simulink model "Combined_electrolyzer_simulink"  (R2022a)
settings: Solver=FixedStepAuto  StartTime=0.0  StopTime=1000  FixedStep=1  RelTol=1e-3
settings Model: Creator=Anupp  LastModifiedBy=Anupp

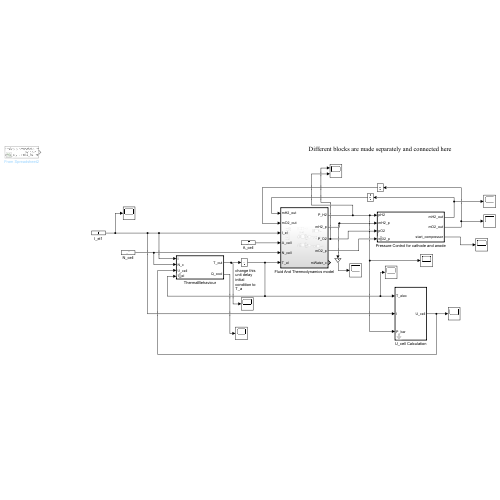
[thumbnail: Simulink's stored preview of the top-level diagram]
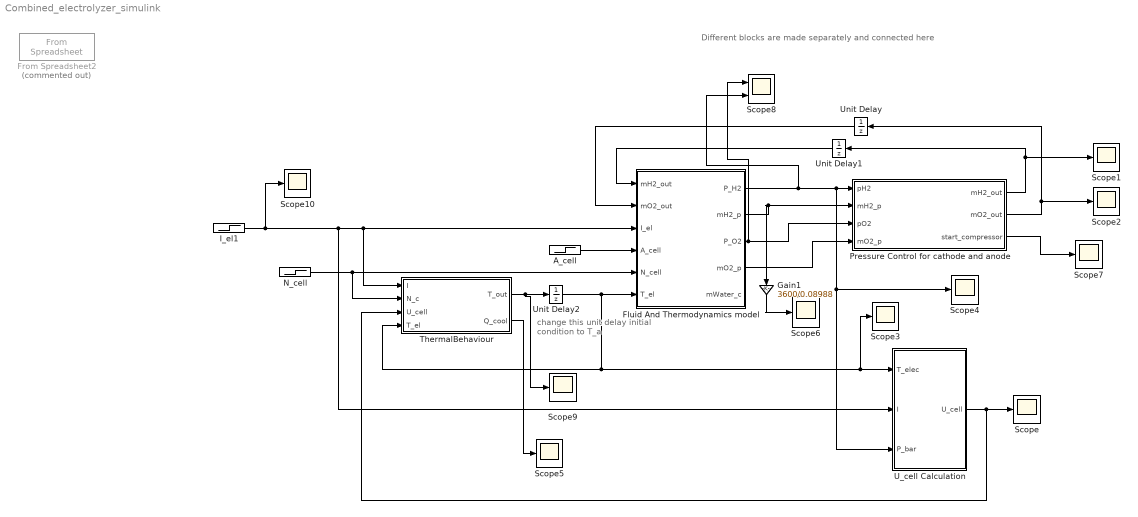
== system Combined_electrolyzer_simulink ==
  note: Different blocks are made separately and connected here
  note: change this unit delay initial condition to T_a
  A_cell : Step  Time=0  After=37.476  SampleTime=0
  Fluid And Thermodynamics model : Subsystem  TreatAsAtomicUnit=on
  From Spreadsheet2 : FromSpreadsheet  Commented=on  FileName=E:\tintan\Matlab alakaline electrolysis new\data test\down_dynamic_halved.csv  SheetName=down_dynamic_halved
  Gain1 : Gain  Gain=3600/0.08988
  I_el1 : Step  Time=0  After=4567.5  SampleTime=0
  N_cell : Step  Time=0  After=326  SampleTime=0
  Pressure Control for cathode and anode : Subsystem  TreatAsAtomicUnit=on  mask{P_nominal=16e+05}
      mask prompts: P_nominal "Nominal Electrolyzer Pressure"
  Scope{,1..7,9..10} (10 alike) : Scope
  Scope8 : Scope  NumInputPorts=2
  ThermalBehaviour : Subsystem  TreatAsAtomicUnit=on  mask{E_tn=1.476, T_a=298, R_t=0.4441, C_t=1.6824e+05, T_nominal=353}
      mask prompts: E_tn "Thermo-neutral voltage (E_tn)"; T_a "Ambient Temperature (kelvin)"; R_t "Thermal Resistance"; C_t "Thermal Capacitance"; T_nominal "Nominal Temperature (kelvin)"
  U_cell Calculation : Subsystem  TreatAsAtomicUnit=on  mask{A=26600, r1=0.8, r2=-0.00763, t1=20, t2=0.1, t3=3.5e+05, s=0.1795, C=0.25}
      mask prompts: A "Area"; r1 "r1 for U_ohm"; r2 "r2 for U_ohm"; t1 "t1 for U_act"; t2 "t2 for U_act"; t3 "t3 for U_act"; s "s for U_act"; C "Concentration by weight (decimal)"
      mask DialogControl DescTextVar Prompt: Put all values in terms in Metres only or Cm only. Also check if U_act variables is for Log or Ln (change accordingly inside the mask). Also, use concentration value as decimal (for eg. use 0.25, don't use 25 percent).
  Unit Delay : UnitDelay  SampleTime=-1  HasFrameUpgradeWarning=on
  Unit Delay1 : UnitDelay  SampleTime=-1  HasFrameUpgradeWarning=on
  Unit Delay2 : UnitDelay  InitialCondition=298  SampleTime=-1  HasFrameUpgradeWarning=on
  wires:
  Fluid And Thermodynamics model/1(P_H2) -> Scope8/2, Scope4/1, U_cell Calculation/3(P_bar), Pressure Control for cathode and anode/1(pH2)
  Fluid And Thermodynamics model/3(P_O2) -> Scope8/1, Pressure Control for cathode and anode/3(pO2)
  Fluid And Thermodynamics model/4(mO2_p) -> Pressure Control for cathode and anode/4(mO2_p)
  Pressure Control for cathode and anode/1(mH2_out) -> Scope1/1, Unit Delay1/1
  Pressure Control for cathode and anode/2(mO2_out) -> Scope2/1, Unit Delay/1
  Unit Delay1/1 -> Fluid And Thermodynamics model/1(mH2_out)
  Unit Delay/1 -> Fluid And Thermodynamics model/2(mO2_out)
  ThermalBehaviour/1(T_out) -> Scope9/1, Unit Delay2/1
  U_cell Calculation/1(U_cell) -> Scope/1, ThermalBehaviour/3(U_cell)
  Unit Delay2/1 -> Scope3/1, U_cell Calculation/1(T_elec), ThermalBehaviour/4(T_el), Fluid And Thermodynamics model/6(T_el)
  I_el1/1 -> U_cell Calculation/2(I), ThermalBehaviour/1(I), Fluid And Thermodynamics model/3(I_el), Scope10/1
  A_cell/1 -> Fluid And Thermodynamics model/4(A_cell)
  N_cell/1 -> ThermalBehaviour/2(N_c), Fluid And Thermodynamics model/5(N_cell)
  ThermalBehaviour/2(Q_cool) -> Scope5/1
  Pressure Control for cathode and anode/3(start_compressor) -> Scope7/1
  Fluid And Thermodynamics model/2(mH2_p) -> Pressure Control for cathode and anode/2(mH2_p), Gain1/1
  Gain1/1 -> Scope6/1

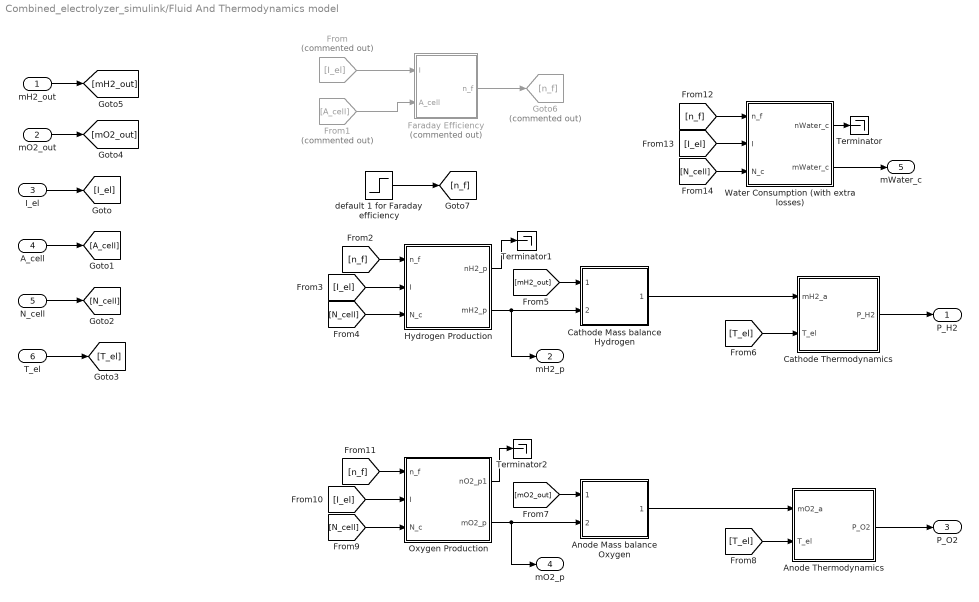
== system Combined_electrolyzer_simulink/Fluid And Thermodynamics model ==
  mH2_out : Inport
  mO2_out : Inport  Port=2
  I_el : Inport  Port=3
  A_cell : Inport  Port=4
  N_cell : Inport  Port=5
  T_el : Inport  Port=6
  Anode Mass balance Oxygen : Subsystem
  Anode Thermodynamics : Subsystem  mask{V=0.001}
      mask prompts: V "Anode Volume"
  Cathode Mass balance Hydrogen : Subsystem
  Cathode Thermodynamics : Subsystem  mask{V=0.001}
      mask prompts: V "Cathode Volume"
  Faraday Efficiency : Subsystem  Commented=on  mask{a1=0, a2=0, a3=0}
      mask DialogControl DescTextVar Prompt: Define Faraday's efficiency parameters for alkaline electrolyser
  From : From  Commented=on  GotoTag=I_el
  From1 : From  Commented=on  GotoTag=A_cell
  Goto6 : Goto  Commented=on  GotoTag=n_f
  Hydrogen Production : Subsystem
  Oxygen Production : Subsystem
  Terminator : Terminator
  Terminator1 : Terminator
  Terminator2 : Terminator
  Water Consumption (with extra losses) : Subsystem
  default 1 for Faraday efficiency : Step  Time=0  After=0.86  SampleTime=0
  P_H2 : Outport
  mH2_p : Outport  Port=2
  P_O2 : Outport  Port=3
  mO2_p : Outport  Port=4
  mWater_c : Outport  Port=5
  wires:
  From1/1 -> Faraday Efficiency/2(A_cell)
  From/1 -> Faraday Efficiency/1(I)
  Cathode Mass balance Hydrogen/1(mH2_a) -> Cathode Thermodynamics/1(mH2_a)
  [n_f] -> Hydrogen Production/1(n_f)
  T_el/1 -> [T_el]
  [I_el] -> Water Consumption (with extra losses)/2(I)
  Hydrogen Production/2(mH2_p) -> mH2_p/1, Cathode Mass balance Hydrogen/2(mH2_p)
  N_cell/1 -> [N_cell]
  I_el/1 -> [I_el]
  [n_f] -> Oxygen Production/1(n_f)
  mO2_out/1 -> [mO2_out]
  Water Consumption (with extra losses)/2(mWater_c) -> mWater_c/1
  A_cell/1 -> [A_cell]
  mH2_out/1 -> [mH2_out]
  [I_el] -> Oxygen Production/2(I)
  [N_cell] -> Oxygen Production/3(N_c)
  [mH2_out] -> Cathode Mass balance Hydrogen/1(mH2_out)
  [N_cell] -> Hydrogen Production/3(N_c)
  Oxygen Production/2(mO2_p) -> mO2_p/1, Anode Mass balance Oxygen/2(mO2_p)
  [I_el] -> Hydrogen Production/2(I)
  Faraday Efficiency/1(n_f) -> Goto6/1
  [T_el] -> Cathode Thermodynamics/2(T_el)
  [N_cell] -> Water Consumption (with extra losses)/3(N_c)
  [n_f] -> Water Consumption (with extra losses)/1(n_f)
  [T_el] -> Anode Thermodynamics/2(T_el)
  Anode Mass balance Oxygen/1(mO2_a) -> Anode Thermodynamics/1(mO2_a)
  [mO2_out] -> Anode Mass balance Oxygen/1(mO2_out)
  Cathode Thermodynamics/1(P_H2) -> P_H2/1
  Anode Thermodynamics/1(P_O2) -> P_O2/1
  Water Consumption (with extra losses)/1(nWater_c) -> Terminator/1
  Hydrogen Production/1(nH2_p) -> Terminator1/1
  Oxygen Production/1(nO2_p1) -> Terminator2/1
  default 1 for Faraday efficiency/1 -> [n_f]

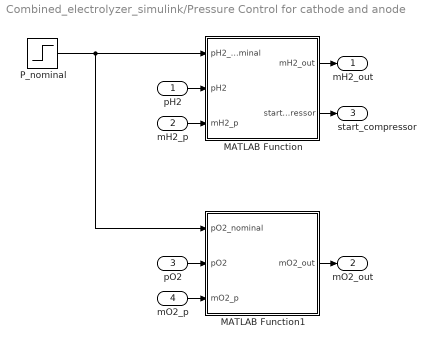
== system Combined_electrolyzer_simulink/Pressure Control for cathode and anode ==
  pH2 : Inport
  mH2_p : Inport  Port=2
  pO2 : Inport  Port=3
  mO2_p : Inport  Port=4
  MATLAB Function : MATLAB Function  TreatAsAtomicUnit=on
  MATLAB Function1 : MATLAB Function  TreatAsAtomicUnit=on
  P_nominal : Step  Time=0  After=P_nominal  SampleTime=0
  mH2_out : Outport
  mO2_out : Outport  Port=2
  start_compressor : Outport  Port=3
  wires:
  P_nominal/1 -> MATLAB Function1/1(pO2_nominal), MATLAB Function/1(pH2_nominal)
  mH2_p/1 -> MATLAB Function/3(mH2_p)
  MATLAB Function/2(start_compressor) -> start_compressor/1
  MATLAB Function/1(mH2_out) -> mH2_out/1
  pH2/1 -> MATLAB Function/2(pH2)
  MATLAB Function1/1(mO2_out) -> mO2_out/1
  mO2_p/1 -> MATLAB Function1/3(mO2_p)
  pO2/1 -> MATLAB Function1/2(pO2)

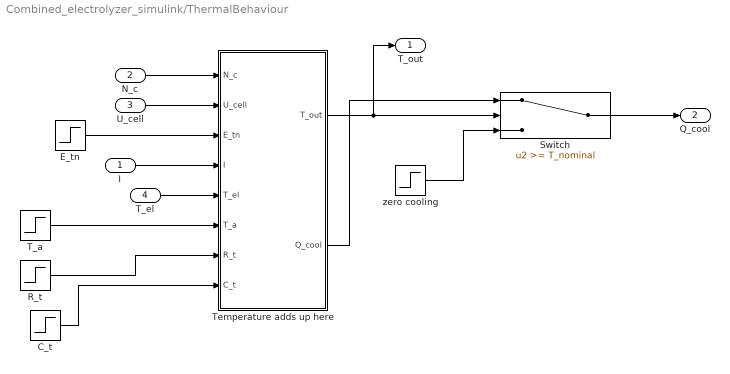
== system Combined_electrolyzer_simulink/ThermalBehaviour ==
  I : Inport
  N_c : Inport  Port=2
  U_cell : Inport  Port=3
  T_el : Inport  Port=4
  C_t : Step  Time=0  After=C_t  SampleTime=0
  E_tn : Step  Time=0  After=E_tn  SampleTime=0
  R_t : Step  Time=0  After=R_t  SampleTime=0
  Switch : Switch  Threshold=T_nominal  SaturateOnIntegerOverflow=off  InputSameDT=off
  T_a : Step  Time=0  After=T_a  SampleTime=0
  Temperature adds up here : Subsystem
  zero cooling : Step  Time=0  After=0  SampleTime=0
  T_out : Outport
  Q_cool : Outport  Port=2
  wires:
  C_t/1 -> Temperature adds up here/8(C_t)
  I/1 -> Temperature adds up here/4(I)
  E_tn/1 -> Temperature adds up here/3(E_tn)
  U_cell/1 -> Temperature adds up here/2(U_cell)
  N_c/1 -> Temperature adds up here/1(N_c)
  T_a/1 -> Temperature adds up here/6(T_a)
  R_t/1 -> Temperature adds up here/7(R_t)
  T_el/1 -> Temperature adds up here/5(T_el)
  Temperature adds up here/1(T_out) -> T_out/1, Switch/2
  zero cooling/1 -> Switch/3
  Switch/1 -> Q_cool/1
  Temperature adds up here/2(Q_cool) -> Switch/1

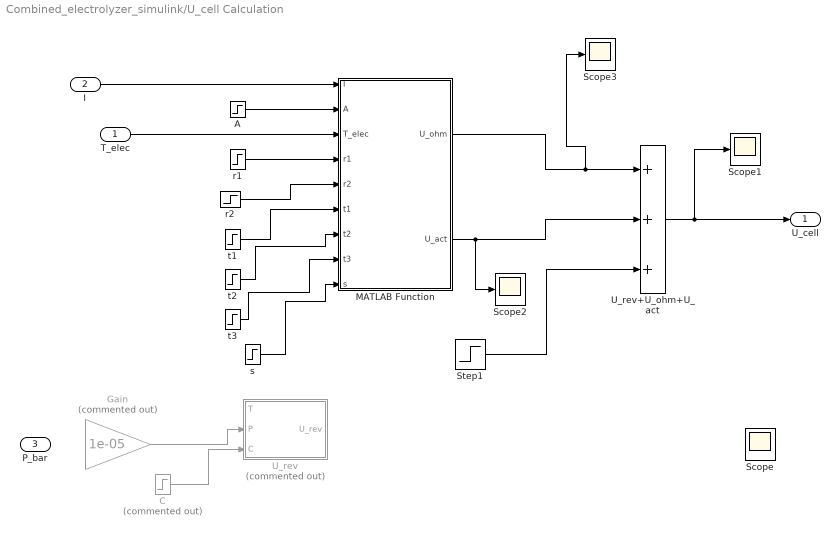
== system Combined_electrolyzer_simulink/U_cell Calculation ==
  T_elec : Inport
  I : Inport  Port=2
  P_bar : Inport  Port=3
  A : Step  Time=0  After=A  SampleTime=0
  C : Step  Commented=on  Time=0  After=C  SampleTime=0
  Gain : Gain  Commented=on  Gain=1e-05
  MATLAB Function : MATLAB Function  TreatAsAtomicUnit=on
  Scope{,1..3} (4 alike) : Scope
  Step1 : Step  Time=0  After=1.2  SampleTime=0
  U_rev : MATLAB Function  Commented=on  TreatAsAtomicUnit=on
  U_rev+U_ohm+U_act : Sum  Inputs=+++
  r1 : Step  Time=0  After=r1  SampleTime=0
  r2 : Step  Time=0  After=r2  SampleTime=0
  s : Step  Time=0  After=s  SampleTime=0
  t1 : Step  Time=0  After=t1  SampleTime=0
  t2 : Step  Time=0  After=t2  SampleTime=0
  t3 : Step  Time=0  After=t3  SampleTime=0
  U_cell : Outport
  wires:
  T_elec/1 -> MATLAB Function/3(T_elec)
  U_rev+U_ohm+U_act/1 -> U_cell/1, Scope1/1
  C/1 -> U_rev/3(C)
  r1/1 -> MATLAB Function/4(r1)
  r2/1 -> MATLAB Function/5(r2)
  t1/1 -> MATLAB Function/6(t1)
  t2/1 -> MATLAB Function/7(t2)
  t3/1 -> MATLAB Function/8(t3)
  s/1 -> MATLAB Function/9(s)
  I/1 -> MATLAB Function/1(I)
  A/1 -> MATLAB Function/2(A)
  MATLAB Function/2(U_act) -> Scope2/1, U_rev+U_ohm+U_act/2
  MATLAB Function/1(U_ohm) -> Scope3/1, U_rev+U_ohm+U_act/1
  Gain/1 -> U_rev/2(P)
  Step1/1 -> U_rev+U_ohm+U_act/3

== system Combined_electrolyzer_simulink/Fluid And Thermodynamics model/Anode Mass balance Oxygen ==
  mO2_out : Inport
  mO2_p : Inport  Port=2
  MATLAB Function : MATLAB Function  TreatAsAtomicUnit=on
  mO2_a : Outport
  wires:
  MATLAB Function/1(mO2_a) -> mO2_a/1
  mO2_p/1 -> MATLAB Function/2(mO2_p)
  mO2_out/1 -> MATLAB Function/1(mO2_out)

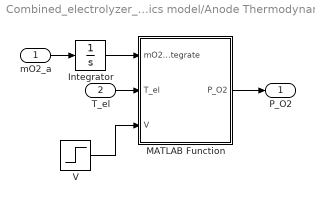
== system Combined_electrolyzer_simulink/Fluid And Thermodynamics model/Anode Thermodynamics ==
  mO2_a : Inport
  T_el : Inport  Port=2
  Integrator : Integrator
  MATLAB Function : MATLAB Function  TreatAsAtomicUnit=on
  V : Step  Time=0  After=V  SampleTime=0
  P_O2 : Outport
  wires:
  T_el/1 -> MATLAB Function/2(T_el)
  mO2_a/1 -> Integrator/1
  Integrator/1 -> MATLAB Function/1(mO2_a_integrate)
  MATLAB Function/1(P_O2) -> P_O2/1
  V/1 -> MATLAB Function/3(V)

== system Combined_electrolyzer_simulink/Fluid And Thermodynamics model/Cathode Mass balance Hydrogen ==
  mH2_out : Inport
  mH2_p : Inport  Port=2
  MATLAB Function : MATLAB Function  TreatAsAtomicUnit=on
  mH2_a : Outport
  wires:
  MATLAB Function/1(mH2_a) -> mH2_a/1
  mH2_p/1 -> MATLAB Function/2(mH2_p)
  mH2_out/1 -> MATLAB Function/1(mH2_out)

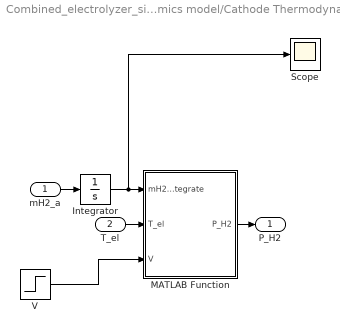
== system Combined_electrolyzer_simulink/Fluid And Thermodynamics model/Cathode Thermodynamics ==
  mH2_a : Inport
  T_el : Inport  Port=2
  Integrator : Integrator
  MATLAB Function : MATLAB Function  TreatAsAtomicUnit=on
  Scope : Scope
  V : Step  Time=0  After=V  SampleTime=0
  P_H2 : Outport
  wires:
  Integrator/1 -> Scope/1, MATLAB Function/1(mH2_a_integrate)
  MATLAB Function/1(P_H2) -> P_H2/1
  mH2_a/1 -> Integrator/1
  T_el/1 -> MATLAB Function/2(T_el)
  V/1 -> MATLAB Function/3(V)

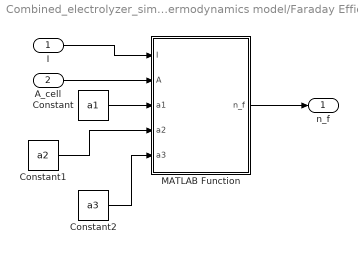
== system Combined_electrolyzer_simulink/Fluid And Thermodynamics model/Faraday Efficiency ==
  I : Inport
  A_cell : Inport  Port=2
  Constant : Constant  Value=a1
  Constant1 : Constant  Value=a2
  Constant2 : Constant  Value=a3
  MATLAB Function : MATLAB Function  TreatAsAtomicUnit=on
  n_f : Outport
  wires:
  MATLAB Function/1(n_f) -> n_f/1
  Constant2/1 -> MATLAB Function/5(a3)
  Constant1/1 -> MATLAB Function/4(a2)
  A_cell/1 -> MATLAB Function/2(A)
  I/1 -> MATLAB Function/1(I)
  Constant/1 -> MATLAB Function/3(a1)

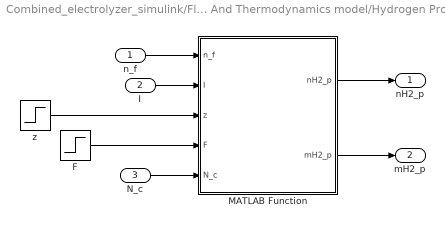
== system Combined_electrolyzer_simulink/Fluid And Thermodynamics model/Hydrogen Production ==
  n_f : Inport
  I : Inport  Port=2
  N_c : Inport  Port=3
  F : Step  Time=0  After=96485  SampleTime=0
  MATLAB Function : MATLAB Function  TreatAsAtomicUnit=on
  z : Step  Time=0  After=2  SampleTime=0
  nH2_p : Outport
  mH2_p : Outport  Port=2
  wires:
  n_f/1 -> MATLAB Function/1(n_f)
  I/1 -> MATLAB Function/2(I)
  MATLAB Function/2(mH2_p) -> mH2_p/1
  N_c/1 -> MATLAB Function/5(N_c)
  F/1 -> MATLAB Function/4(F)
  z/1 -> MATLAB Function/3(z)
  MATLAB Function/1(nH2_p) -> nH2_p/1

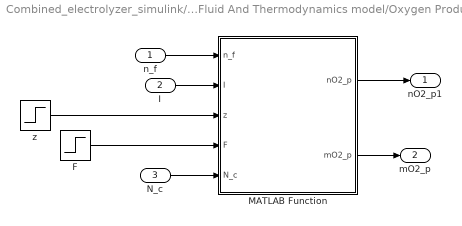
== system Combined_electrolyzer_simulink/Fluid And Thermodynamics model/Oxygen Production ==
  n_f : Inport
  I : Inport  Port=2
  N_c : Inport  Port=3
  F : Step  Time=0  After=96485  SampleTime=0
  MATLAB Function : MATLAB Function  TreatAsAtomicUnit=on
  z : Step  Time=0  After=2  SampleTime=0
  nO2_p1 : Outport
  mO2_p : Outport  Port=2
  wires:
  n_f/1 -> MATLAB Function/1(n_f)
  I/1 -> MATLAB Function/2(I)
  MATLAB Function/2(mO2_p) -> mO2_p/1
  N_c/1 -> MATLAB Function/5(N_c)
  MATLAB Function/1(nO2_p) -> nO2_p1/1
  F/1 -> MATLAB Function/4(F)
  z/1 -> MATLAB Function/3(z)

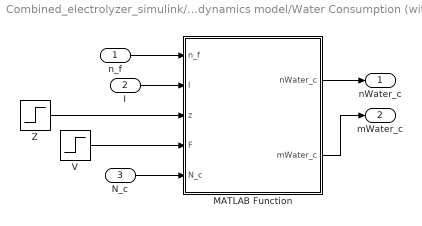
== system Combined_electrolyzer_simulink/Fluid And Thermodynamics model/Water Consumption (with extra losses) ==
  n_f : Inport
  I : Inport  Port=2
  N_c : Inport  Port=3
  MATLAB Function : MATLAB Function  TreatAsAtomicUnit=on
  V : Step  Time=0  After=96485  SampleTime=0
  Z : Step  Time=0  After=2  SampleTime=0
  nWater_c : Outport
  mWater_c : Outport  Port=2
  wires:
  n_f/1 -> MATLAB Function/1(n_f)
  I/1 -> MATLAB Function/2(I)
  MATLAB Function/2(mWater_c) -> mWater_c/1
  N_c/1 -> MATLAB Function/5(N_c)
  MATLAB Function/1(nWater_c) -> nWater_c/1
  Z/1 -> MATLAB Function/3(z)
  V/1 -> MATLAB Function/4(F)

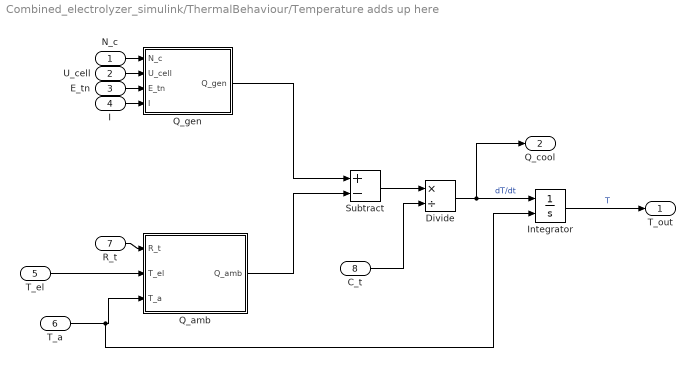
== system Combined_electrolyzer_simulink/ThermalBehaviour/Temperature adds up here ==
  N_c : Inport
  U_cell : Inport  Port=2
  E_tn : Inport  Port=3
  I : Inport  Port=4
  T_el : Inport  Port=5
  T_a : Inport  Port=6
  R_t : Inport  Port=7
  C_t : Inport  Port=8
  Divide : Product  Inputs=*/
  Integrator : Integrator  InitialConditionSource=external  LimitOutput=on  UpperSaturationLimit=T_nominal
  Q_amb : MATLAB Function  TreatAsAtomicUnit=on
  Q_gen : MATLAB Function  TreatAsAtomicUnit=on
  Subtract : Sum  Inputs=+-
  T_out : Outport
  Q_cool : Outport  Port=2
  wires:
  Q_gen/1(Q_gen) -> Subtract/1
  Q_amb/1(Q_amb) -> Subtract/2
  Integrator/1 -> T_out/1  "T"
  Divide/1 -> Q_cool/1, Integrator/1  "dT/dt"
  C_t/1 -> Divide/2
  R_t/1 -> Q_amb/1(R_t)
  Subtract/1 -> Divide/1
  N_c/1 -> Q_gen/1(N_c)
  E_tn/1 -> Q_gen/3(E_tn)
  I/1 -> Q_gen/4(I)
  U_cell/1 -> Q_gen/2(U_cell)
  T_a/1 -> Integrator/2, Q_amb/3(T_a)
  T_el/1 -> Q_amb/2(T_el)

== matlab function Combined_electrolyzer_simulink/Fluid And Thermodynamics model/Cathode Thermodynamics/MATLAB Function ==
  data: mH2_a_integrate input; P_H2 output; T_el input; V input
function P_H2 = fcn(mH2_a_integrate,T_el, V)

P_H2 =  (8.3143 * T_el)/(V*2.016*(1e-3)) * mH2_a_integrate;

end

== matlab function Combined_electrolyzer_simulink/Fluid And Thermodynamics model/Faraday Efficiency/MATLAB Function ==
  data: I input; n_f output; A input; a1 input; a2 input; a3 input
function n_f = fcn(I,A,a1,a2,a3)

n_f = a1 .* exp(a2/(I/A) + a3/(I/A)^2);

end

== matlab function Combined_electrolyzer_simulink/Fluid And Thermodynamics model/Hydrogen Production/MATLAB Function ==
  data: nH2_p output; n_f input; mH2_p output; I input; z input; F input; N_c input
function [nH2_p,mH2_p] = fcn(n_f,I,z,F,N_c)

nH2_p = n_f * I * N_c / (z * F);
mH2_p = 2.016 * 1e-3 * nH2_p; 

end

== matlab function Combined_electrolyzer_simulink/Fluid And Thermodynamics model/Oxygen Production/MATLAB Function ==
  data: nO2_p output; n_f input; mO2_p output; I input; z input; F input; N_c input
function [nO2_p,mO2_p] = fcn(n_f,I,z,F,N_c)

nO2_p = 0.5 * n_f * I * N_c / (z * F);

mO2_p = 32 * 1e-3 * nO2_p;

end

== matlab function Combined_electrolyzer_simulink/Fluid And Thermodynamics model/Water Consumption (with extra losses)/MATLAB Function ==
  data: nWater_c output; n_f input; mWater_c output; I input; z input; F input; N_c input
function [nWater_c,mWater_c] = fcn(n_f,I,z,F,N_c)

nWater_c = 1.25 * n_f * I * N_c / (z * F);

mWater_c = 18.015 * 1e-3 * nWater_c;

end

== matlab function Combined_electrolyzer_simulink/ThermalBehaviour/Temperature adds up here/Q_gen ==
  data: N_c input; Q_gen output; U_cell input; E_tn input; I input
function Q_gen = fcn(N_c,U_cell,E_tn,I)

Q_gen = N_c * (U_cell - E_tn) * I;

end

== matlab function Combined_electrolyzer_simulink/U_cell Calculation/MATLAB Function ==
  data: I input; U_ohm output; A input; T_elec input; r1 input; r2 input; t1 input; t2 input; t3 input; s input; U_act output
function [U_ohm, U_act] = fcn(I,A,T_elec,r1,r2,t1,t2,t3,s)

T = T_elec-273;

i = I/A;

U_ohm = (r1 + r2*T)*i;

U_act = s*log((t1 + t2/T + t3/(T^2))*i + 1);

end

== matlab function Combined_electrolyzer_simulink/ThermalBehaviour/Temperature adds up here/Q_amb ==
  data: R_t input; Q_amb output; T_el input; T_a input
function Q_amb = fcn(R_t,T_el,T_a)

Q_amb = (T_el - T_a)/R_t;

end

== matlab function Combined_electrolyzer_simulink/U_cell Calculation/U_rev ==
  data: T input; U_rev output; P input; C input
function U_rev = fcn(T,P,C)
% T = 398;
% P = 9.44;
% C = 0.25;
R = 8.3144598; %J. mol-1
z = 2; %of hydrogen is used, don't know why oxygen is not used
F = 96485; %Faradays constant C/mol
M = ((312500/17533)*C)/(1-C); %molality

U_0rev = 1.5184-1.5421*10^(-3)*T+9.526*10^(-5)*T*log(T)+9.84*10^(-8)*(T)^2;

a = -0.0151*M - 1.6788*10^(-3)*(M^2)+2.2588*10^(-5)*(M^3);
b = 1-1.2062*10^(-3)*M+5.6024*10^(-4)*(M^2)-7.8228*10^(-6)*(M^3);
P_vH2O = 10^(5.1962-(1730.63/(233.426+T-273)));
%P_vH2O = exp(81.6179 - 7699.68/T - 10.9*log(T) + 9.5891 * 10^(-3) * T);

P_vKOH = exp(2.302*a+b*log(P_vH2O));

a_H2O_KOH = exp(-0.05192*M+0.003302*(M^2)+((3.177*M-2.131*(M^2))/T));

U_rev = U_0rev + ((R*T)/(z*F))*log10(((P-P_vKOH)*((P-P_vKOH)^0.5))/(a_H2O_KOH));

end

== matlab function Combined_electrolyzer_simulink/Pressure Control for cathode and anode/MATLAB Function ==
  data: pH2_nominal input; mH2_out output; pH2 input; mH2_p input; start_compressor output
function [mH2_out,start_compressor]  = fcn(pH2_nominal,pH2,mH2_p)

    if pH2 >= pH2_nominal
        mH2_out = mH2_p;
        start_compressor = 1;
    else
        mH2_out = 0;
        start_compressor = 0;
    end
end

== matlab function Combined_electrolyzer_simulink/Pressure Control for cathode and anode/MATLAB Function1 ==
  data: pO2_nominal input; mO2_out output; pO2 input; mO2_p input
function mO2_out  = fcn(pO2_nominal,pO2,mO2_p)

    if pO2 >= pO2_nominal
        mO2_out = mO2_p;
    else
        mO2_out = 0;
    end
end

== matlab function Combined_electrolyzer_simulink/Fluid And Thermodynamics model/Anode Mass balance Oxygen/MATLAB Function ==
  data: mO2_out input; mO2_a output; mO2_p input
function mO2_a  = fcn(mO2_out,mO2_p)

mO2_a = mO2_p - mO2_out;

end

== matlab function Combined_electrolyzer_simulink/Fluid And Thermodynamics model/Anode Thermodynamics/MATLAB Function ==
  data: mO2_a_integrate input; P_O2 output; T_el input; V input
function P_O2 = fcn(mO2_a_integrate,T_el, V)

P_O2 =  (8.3143 * T_el)/(V*32*(1e-3)) * mO2_a_integrate;

end

== matlab function Combined_electrolyzer_simulink/Fluid And Thermodynamics model/Cathode Mass balance Hydrogen/MATLAB Function ==
  data: mH2_out input; mH2_a output; mH2_p input
function mH2_a  = fcn(mH2_out,mH2_p)

mH2_a = mH2_p - mH2_out;

end
